simulink model "Desgin_Power_Circuit"  (R2023b)
settings: Solver=VariableStepAuto  StartTime=0.0  StopTime=0.3  RelTol=1e-3
libraries: spsDiodeLib x5, spsVoltageMeasurementLib x5, spsCurrentMeasurementLib x4, spsMeanLib x3, spsSeriesRLCBranchLib x3, spsTHDLib x2, spsACVoltageSourceLib x1, spsMosfetLib x1, slpidlib x1, simulink_extras x1, spsPowerLib x1, sps_lib x1
settings Model: Creator=HP  LastModifiedBy=HP

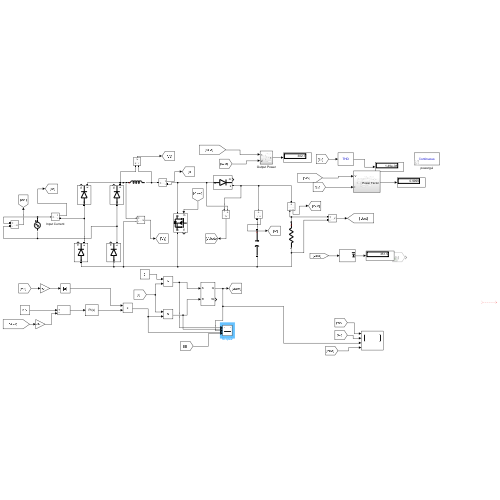
[thumbnail: Simulink's stored preview of the top-level diagram]
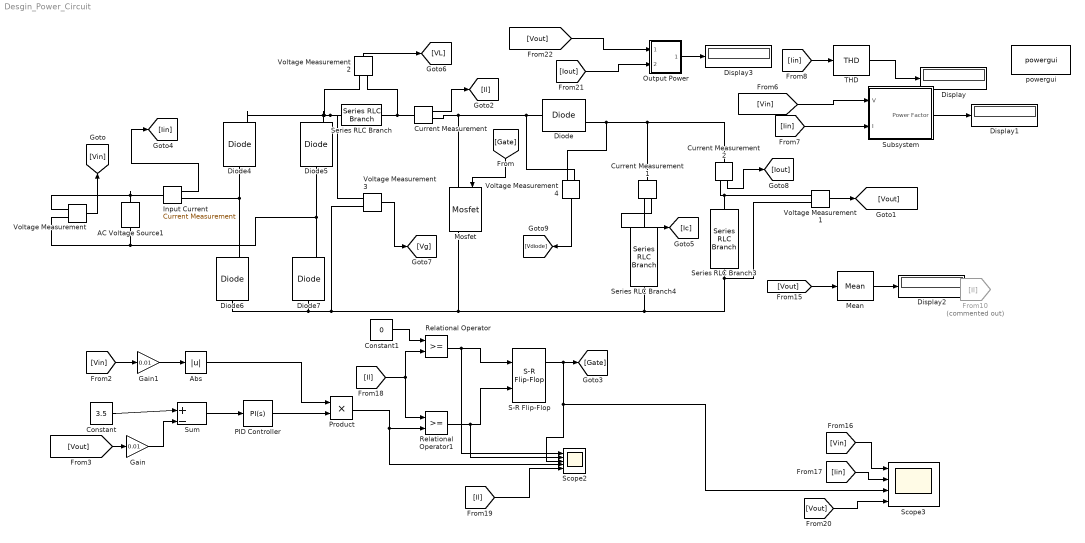
== system Desgin_Power_Circuit ==
  AC Voltage Source1 : spsACVoltageSourceLib/AC Voltage Source  Amplitude=220*sqrt(2)  Phase=0  Frequency=50  SampleTime=0  Measurements=None  BusType=swing  Pref=10e3  Qref=0  Qmin=-inf  Qmax=+inf
  Abs : Abs  SaturateOnIntegerOverflow=off
  Constant : Constant  Value=3.5
  Constant1 : Constant  Value=0
  Current Measurement : spsCurrentMeasurementLib/Current Measurement  PhasorSimulation=off  OutputType=Complex  PSBequivalent=0
  Current Measurement1 : spsCurrentMeasurementLib/Current Measurement  PhasorSimulation=off  OutputType=Complex  PSBequivalent=0
  Current Measurement2 : spsCurrentMeasurementLib/Current Measurement  PhasorSimulation=off  OutputType=Complex  PSBequivalent=0
  Diode{,4..7} (5 alike) : spsDiodeLib/Diode  Ron=0.001  Lon=0  Vf=0.8  IC=0  UseSnubber=0  Rs=500  Cs=250e-9  Measurements=on
  Display{,1..3} (4 alike) : Display
  From10 : From  Commented=on  GotoTag=Il
  Gain : Gain  Gain=0.01
  Gain1 : Gain  Gain=0.01
  Input Current : spsCurrentMeasurementLib/Current Measurement  PhasorSimulation=off  OutputType=Complex  PSBequivalent=0
  Mean : spsMeanLib/Mean  Freq=60  Vinit=0  Ts=0
  Mosfet : spsMosfetLib/Mosfet  Ron=0.1  Lon=0  Rd=0.01  Vfd=0  IC=0  Rs=1e5  Cs=inf  Measurements=on
  Output Power : Subsystem
  PID Controller : slpidlib/PID Controller  Controller=PI  Form=Parallel  TimeDomain=Continuous-time  UseExternalTs=off  SampleTime=-1  IntegratorMethod=Forward Euler  FilterMethod=Forward Euler  ControllerParametersSource=internal  P=0.4  I=25  UseKiTs=off  D=0  N=100  UseFilter=on  TunerSelectOption=Frequency Response Based  InitialConditionSource=internal  InitialConditionForIntegrator=0  InitialConditionForFilter=0  DifferentiatorICPrevScaledInput=0  ExternalReset=none  TrackingMode=off  Kt=1  LimitOutput=off  SatLimitsSource=internal  UpperSaturationLimit=inf  LowerSaturationLimit=-inf  LinearizeAsGain=on  AntiWindupMode=none  Kb=1  LimitIntegrator=off  UpperIntegratorSaturationLimit=inf  LowerIntegratorSaturationLimit=-inf  POutMin=[]  POutMax=[]  IOutMin=[]  IOutMax=[]  DOutMin=[]  DOutMax=[]  NOutMin=[]  NOutMax=[]  SumOutMin=[]  SumOutMax=[]  SaturationOutMin=[]  SaturationOutMax=[]  PParamMin=[]  PParamMax=[]  IParamMin=[]  IParamMax=[]  DParamMin=[]  DParamMax=[]  NParamMin=[]  NParamMax=[]  KbParamMin=[]  KbParamMax=[]  KtParamMin=[]  KtParamMax=[]  KbOutMin=[]  KbOutMax=[]  KtOutMin=[]  KtOutMax=[]  IntegratorOutMin=[]  IntegratorOutMax=[]  FilterOutMin=[]  FilterOutMax=[]  SumI1OutMin=[]  SumI1OutMax=[]  SumI2OutMin=[]  SumI2OutMax=[]  SumI3OutMin=[]  SumI3OutMax=[]  SumI4OutMin=[]  SumI4OutMax=[]  SumDOutMin=[]  SumDOutMax=[]  DifferentiatorOutMin=[]  DifferentiatorOutMax=[]  FilterDiffOutCoefMin=[]  FilterDiffOutCoefMax=[]  ReciprocalOutMin=[]  ReciprocalOutMax=[]  SumDenOutMin=[]  SumDenOutMax=[]  SumNumOutMin=[]  SumNumOutMax=[]  DivideOutMin=[]  DivideOutMax=[]  UdiffTsProdOutMin=[]  UdiffTsProdOutMax=[]  NTsProdOutMin=[]  NTsProdOutMax=[]  UintegralTsProdOutMin=[]  UintegralTsProdOutMax=[]  UngainTsProdOutMin=[]  UngainTsProdOutMax=[]  ClampingZeroOutDataTypeStr=Inherit: Inherit via back propagation  ClampingZeroOutMin=[]  ClampingZeroOutMax=[]  FilterDenConstantOutDataTypeStr=Inherit: Inherit via back propagation  FilterDenConstantOutMin=[]  FilterDenConstantOutMax=[]  PCopyOutDataTypeStr=Inherit: Inherit via back propagation  PCopyOutMin=[]  PCopyOutMax=[]  NCopyOutDataTypeStr=Inherit: Inherit via back propagation  NCopyOutMin=[]  NCopyOutMax=[]  IntegratorContinuousStateAttributes=''  IntegratorStateMustResolveToSignalObject=off  IntegratorRTWStateStorageClass=Auto  FilterContinuousStateAttributes=''  FilterStateMustResolveToSignalObject=off  FilterRTWStateStorageClass=Auto  ParallelPVariant=InternalParameters  IdealPVariant=Disabled  IVariant=InternalParameters  DVariant=Disabled  IntegratorVariant=Continuous  SatVariant=Disabled  AWVariant=Passthrough  PCopyVariant=Disabled  TRVariant=Disabled  FdbkBlocksVariant=Forward  IdealPFdbkVariant=Disabled  SatFdbkVariant=Disabled  DerivativeFilterVariant=Disabled  NVariant=Disabled  NCopyVariant=Disabled_SignalSpec  FilterICVariant=Disabled  IntegratorICVariant=InternalICs  ExternalResetVariant=Disabled  TRSumVariant=Passthrough  SumFdbkVariant=Disabled  SumVariant=Sum_PI  TsampFilterVariant=InternalTs  TsampNgainVariant=Passthrough  TsampIntegralVariant=Disabled_SignalSpec  ExternalSaturationOutDataTypeStr=Inherit: Same as second input
  Product : Product
  Relational Operator : RelationalOperator  OutDataTypeStr=boolean  RndMeth=Simplest  InputSameDT=off
  Relational Operator1 : RelationalOperator  OutDataTypeStr=boolean  RndMeth=Simplest  InputSameDT=off
  S-R Flip-Flop : simulink_extras/Flip Flops/S-R Flip-Flop  initial_condition=1
  Scope2 : Scope  NumInputPorts=5
  Scope3 : Scope  NumInputPorts=4
  Series RLC Branch : spsSeriesRLCBranchLib/Series RLC Branch  LConnTagsString=__new0  RConnTagsString=__new0  BranchType=L  Resistance=1  Inductance=0.342e-3  SetiL0=off  InitialCurrent=0  Capacitance=1e-6  Setx0=off  InitialVoltage=0  Measurements=None
  Series RLC Branch3 : spsSeriesRLCBranchLib/Series RLC Branch  LConnTagsString=__new0  RConnTagsString=__new0  BranchType=R  Resistance=408  Inductance=1e-3  SetiL0=off  InitialCurrent=0  Capacitance=1e-6  Setx0=off  InitialVoltage=0  Measurements=None
  Series RLC Branch4 : spsSeriesRLCBranchLib/Series RLC Branch  LConnTagsString=__new0  RConnTagsString=__new0  BranchType=C  Resistance=1  Inductance=1e-3  SetiL0=off  InitialCurrent=0  Capacitance=150e-6  Setx0=off  InitialVoltage=350  Measurements=None
  Subsystem : Subsystem
  Sum : Sum  Inputs=|+-
  THD : spsTHDLib/THD  Freq=60  Ts=0
  Voltage Measurement{,1..4} (5 alike) : spsVoltageMeasurementLib/Voltage Measurement  PhasorSimulation=off  OutputType=Complex  PSBequivalent=0
  powergui : sps_lib/powergui  Priority=1  SimulationMode=Continuous  SampleTime=1e-07  frequency=60  Iterations=50  frequencyindice=50  Pbase=100e6  ErrMax=1e-4  UnitsV=kV  UnitsW=MW  buscounter=0  FunctionMessages=off  echomessages=off  EnableUseOfTLC=off  CurrentSourceSwitches=off  DisableSnubberDevices=on  DisableRonSwitches=off  DisableVfSwitches=on  DisplayEquations=on  AutomaticDiscreteSolvers=off  SolverType=Tustin/Backward Euler (TBE)  Interpol=off  ExternalGateDelay=off  methode=off  Ts=100  x0status=blocks  SPID=on  SwTol=0  HookPort=off  NonlinearTolerance=1e-4  nMaxIteration=100  ContinueOnMaxIteration=off  RestoreLinks=warning  ResistiveCurrentMeasurement=off  Frange=[0:2:500]  Ylog=off  Xlog=on  ShowGrid=off  save=off  variable=ZData  structure=0  ZoomFFT=off  StartTime=0.0  cycles=1  DisplayStyle=1  fundamental=60  FreqAxis=off  MaxFrequency=1000  frequencyindicesteady=1  RmsSteady=1  display=off
  wires:
  [Vin] -> Subsystem/1(V)
  Sum/1 -> PID Controller/1
  Relational Operator1/1 -> Scope2/2, S-R Flip-Flop/2
  Mean/1 -> Display2/1
  [Iin] -> Subsystem/2(I)
  [Vin] -> Scope3/1
  Voltage Measurement/1 -> [Vin]
  [Iin] -> THD/1
  Constant/1 -> Sum/1
  ? -> ?
  Current Measurement1/1 -> [Ic]
  [Vout] -> Mean/1
  Input Current/1 -> [Iin]
  [Gate] -> Mosfet/1
  S-R Flip-Flop/1 -> Scope3/3, Scope2/3, [Gate]
  Subsystem/1(Power Factor) -> Display1/1
  [Il] -> Scope2/5
  Relational Operator/1 -> Scope2/1, S-R Flip-Flop/1
  Gain/1 -> Sum/2
  [Vin] -> Gain1/1
  Gain1/1 -> Abs/1
  [Iin] -> Scope3/2
  Current Measurement/1 -> [Il]
  [Vout] -> Gain/1
  PID Controller/1 -> Product/2
  Product/1 -> Scope2/4, Relational Operator1/2
  Voltage Measurement2/1 -> [VL]
  Abs/1 -> Product/1
  Voltage Measurement1/1 -> [Vout]
  Constant1/1 -> Relational Operator/1
  THD/1 -> Display/1
  Voltage Measurement3/1 -> [Vg]
  [Il] -> Relational Operator/2, Relational Operator1/1
  [Vout] -> Scope3/4
  Current Measurement2/1 -> [Iout]
  [Iout] -> Output Power/2(In2)
  [Vout] -> Output Power/1(In1)
  Voltage Measurement4/1 -> [Vdiode]
  Output Power/1(Out1) -> Display3/1
  connections:
  Current Measurement1/LConn1 -- Voltage Measurement4/LConn2 -- Diode/RConn1 -- Current Measurement2/LConn1
  Diode5/RConn1 -- Diode4/RConn1 -- Voltage Measurement3/LConn1 -- Series RLC Branch/LConn1 -- Voltage Measurement2/LConn1
  Series RLC Branch4/RConn1 -- Voltage Measurement1/LConn2 -- Series RLC Branch3/RConn1 -- Mosfet/RConn1 -- Voltage Measurement3/LConn2 -- Diode7/LConn1 -- Diode6/LConn1
  Diode6/RConn1 -- Input Current/RConn1 -- Diode4/LConn1
  Series RLC Branch/RConn1 -- Current Measurement/LConn1 -- Voltage Measurement2/LConn2
  Diode7/RConn1 -- AC Voltage Source1/LConn1 -- Voltage Measurement/LConn2 -- Diode5/LConn1
  Mosfet/LConn1 -- Voltage Measurement4/LConn1 -- Diode/LConn1 -- Current Measurement/RConn1
  Voltage Measurement/LConn1 -- AC Voltage Source1/RConn1 -- Input Current/LConn1
  Current Measurement1/RConn1 -- Series RLC Branch4/LConn1
  Current Measurement2/RConn1 -- Voltage Measurement1/LConn1 -- Series RLC Branch3/LConn1

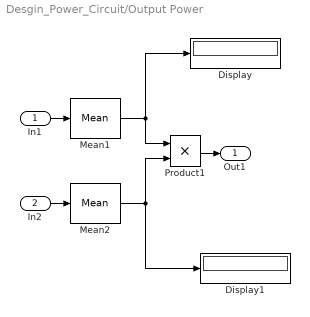
== system Desgin_Power_Circuit/Output Power ==
  In1 : Inport
  In2 : Inport  Port=2
  Display : Display
  Display1 : Display
  Mean1 : spsMeanLib/Mean  Freq=60  Vinit=0  Ts=0
  Mean2 : spsMeanLib/Mean  Freq=60  Vinit=0  Ts=0
  Product1 : Product
  Out1 : Outport
  wires:
  Mean1/1 -> Display/1, Product1/1
  Mean2/1 -> Display1/1, Product1/2
  Product1/1 -> Out1/1
  In2/1 -> Mean2/1
  In1/1 -> Mean1/1

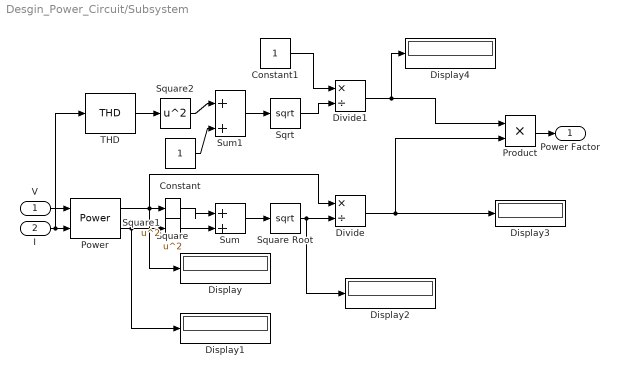
== system Desgin_Power_Circuit/Subsystem ==
  V : Inport
  I : Inport  Port=2
  Constant : Constant  SampleTime=-1
  Constant1 : Constant  SampleTime=-1
  Display{,1..4} (5 alike) : Display
  Divide : Product  Inputs=*/
  Divide1 : Product  Inputs=*/
  Power : spsPowerLib/Power  Freq=50  Vinit=[1, 0]  Iinit=[1, 0]  Ts=0
  Product : Product
  Sqrt : Sqrt
  Square : Math  Operator=square
  Square Root : Sqrt
  Square1 : Math  Operator=square
  Square2 : Math  Operator=square
  Sum : Sum  Inputs=|++
  Sum1 : Sum  Inputs=|++
  THD : spsTHDLib/THD  Freq=60  Ts=0
  Power Factor : Outport
  wires:
  Square/1 -> Sum/1
  Power/1 -> Divide/1, Display/1, Square/1
  Sum/1 -> Square Root/1
  Square Root/1 -> Divide/2, Display2/1
  Square1/1 -> Sum/2
  Power/2 -> Display1/1, Square1/1
  V/1 -> Power/1
  I/1 -> THD/1, Power/2
  Divide/1 -> Display3/1, Product/2
  Product/1 -> Power Factor/1
  THD/1 -> Square2/1
  Square2/1 -> Sum1/1
  Constant/1 -> Sum1/2
  Constant1/1 -> Divide1/1
  Sum1/1 -> Sqrt/1
  Sqrt/1 -> Divide1/2
  Divide1/1 -> Display4/1, Product/1
